simulink model "InvertedPendulumWithLinealization"  (R2017a)
settings: Solver=VariableStepAuto  StartTime=0.0  StopTime=100  RelTol=1e-3
settings Model: Creator=aposad31  LastModifiedBy=Asus

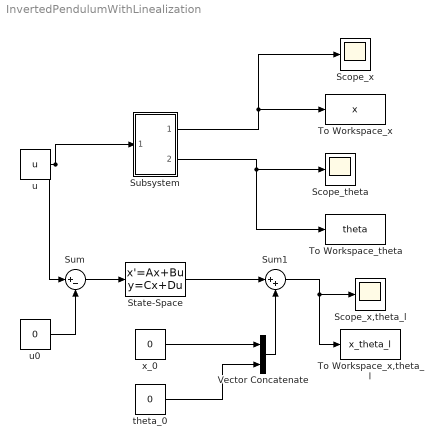
== system InvertedPendulumWithLinealization ==
  Scope_theta : Scope
  Scope_x : Scope
  Scope_x,theta_l : Scope
  State-Space : StateSpace  A=[0 1 0 0; 0 -2/11 147/55 0; 0 0 0 1; 0 5/11 -343/11 0]  B=[0; 20/11; 0; -50/11]  C=[1 0 0 0; 0 0 1 0]  D=[0; 0]  X0=0
  Subsystem : Subsystem  mask{M=0.5, m_p=0.2, b=0.1, L=0.3, I=0.006, g=9.8, dx0=0, d2x0=0, dtheta0=0, d2theta0=0}
      mask prompts: m_p "m"
      mask TypeOptions M: M/Value
      mask TypeOptions m_p: m/Value
      mask TypeOptions b: b/Value
      mask TypeOptions L: L/Value
      mask TypeOptions I: I/Value
      mask TypeOptions g: g/Value
      mask TypeOptions dx0: dx/InitialCondition
      mask TypeOptions d2x0: d2x/InitialCondition
      mask TypeOptions dtheta0: dtheta/InitialCondition
      mask TypeOptions d2theta0: d2theta/InitialCondition
  Sum : Sum  Inputs=|+-
  Sum1 : Sum  Inputs=|++
  To Workspace_theta : ToWorkspace  VariableName=theta  SaveFormat=Timeseries  SampleTime=-1
  To Workspace_x : ToWorkspace  VariableName=x  SaveFormat=Timeseries  SampleTime=-1
  To Workspace_x,theta_l : ToWorkspace  VariableName=x_theta_l  SaveFormat=Timeseries  SampleTime=-1
  Vector Concatenate : Concatenate
  theta_0 : Constant  Value=0
  u : Constant  Value=u
  u0 : Constant  Value=0
  x_0 : Constant  Value=0
  wires:
  Sum/1 -> State-Space/1
  u0/1 -> Sum/2
  State-Space/1 -> Sum1/1
  Vector Concatenate/1 -> Sum1/2
  theta_0/1 -> Vector Concatenate/2
  x_0/1 -> Vector Concatenate/1
  Sum1/1 -> To Workspace_x,theta_l/1, Scope_x,theta_l/1
  u/1 -> Sum/1, Subsystem/1(In3)
  Subsystem/1(Out1) -> Scope_x/1, To Workspace_x/1
  Subsystem/2(Out2) -> Scope_theta/1, To Workspace_theta/1

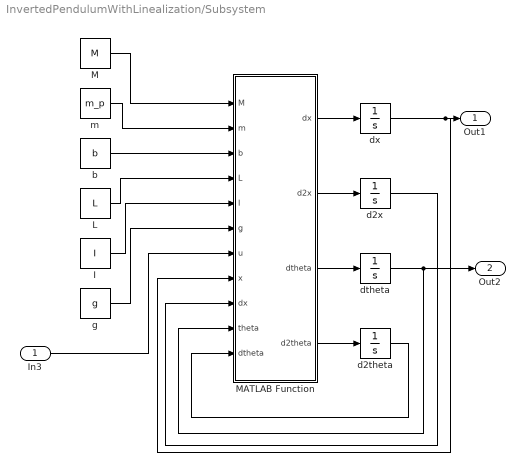
== system InvertedPendulumWithLinealization/Subsystem ==
  In3 : Inport
  I : Constant  Value=I
  L : Constant  Value=L
  M : Constant  Value=M
  MATLAB Function : MATLAB Function  TreatAsAtomicUnit=on
  b : Constant  Value=b
  d2theta : Integrator  InitialCondition=d2theta0
  d2x : Integrator  InitialCondition=d2x0
  dtheta : Integrator  InitialCondition=dtheta0
  dx : Integrator  InitialCondition=dx0
  g : Constant  Value=g
  m : Constant  Value=m_p
  Out1 : Outport
  Out2 : Outport  Port=2
  wires:
  dx/1 -> MATLAB Function/8(x), Out1/1
  MATLAB Function/2(d2x) -> d2x/1
  In3/1 -> MATLAB Function/7(u)
  m/1 -> MATLAB Function/2(m)
  MATLAB Function/1(dx) -> dx/1
  dtheta/1 -> MATLAB Function/10(theta), Out2/1
  d2theta/1 -> MATLAB Function/11("dtheta ")
  MATLAB Function/3(dtheta) -> dtheta/1
  M/1 -> MATLAB Function/1(M)
  b/1 -> MATLAB Function/3(b)
  MATLAB Function/4(d2theta) -> d2theta/1
  d2x/1 -> MATLAB Function/9("dx ")
  g/1 -> MATLAB Function/6(g)
  L/1 -> MATLAB Function/4(L)
  I/1 -> MATLAB Function/5(I)

== matlab function InvertedPendulumWithLinealization/Subsystem/MATLAB Function ==
  data: M input; m input; b input; L input; I input; g input; u input; dx output; x input; dx input; theta input; dtheta input; d2x output; dtheta output; d2theta output
function [dx, d2x, dtheta, d2theta] = fcn(M, m, b, L, I, g, u, x, dx, theta, dtheta)
    denominator = (M+m)*(I+m*L^2)-m^2*L^2*cos(theta)^2;
    dx = dx;
    d2x = ((I+m*L^2)*(u-b*dx+m*L*dtheta^2*sin(theta))+m^2*L^2*g*sin(theta)*cos(theta))/denominator;
    dtheta = dtheta;
    d2theta = (-m*L*u*cos(theta)+m*L*b*dx*cos(theta)-m^2*L^2*dtheta^2*sin(theta)*cos(theta)-(M+m)*m*g*L*sin(theta))/denominator;
end
